simulink model "ForceBasedRollCenterModel"  (R2020b)
settings: Solver=VariableStepAuto  StartTime=0.0  StopTime=10.0  MaxStep=10E-2  RelTol=1e-3
settings Model: Creator=Authorized User  LastModifiedBy=Authorized User

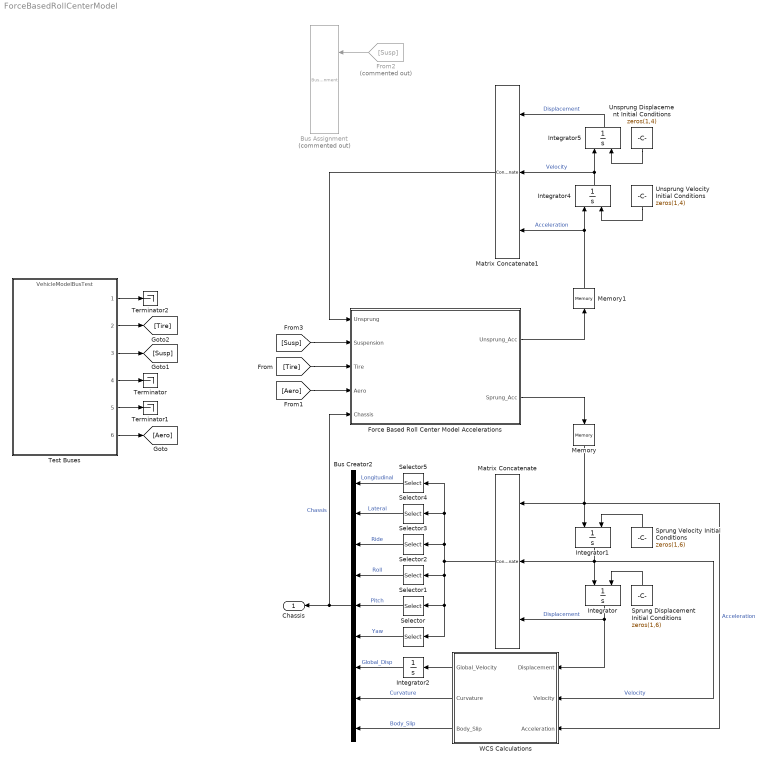
== system ForceBasedRollCenterModel ==
  Bus Assignment : BusAssignment  Commented=on  AssignedSignals=signal1
  Bus Creator2 : BusCreator  Inputs=9
  Force Based Roll Center Model Accelerations : MATLAB Function  TreatAsAtomicUnit=on
  From2 : From  Commented=on  GotoTag=Susp
  Integrator{,1,4..5} (4 alike) : Integrator  InitialConditionSource=external
  Integrator2 : Integrator
  Matrix Concatenate : Concatenate  NumInputs=3  Mode=Multidimensional array  ConcatenateDimension=2
  Matrix Concatenate1 : Concatenate  NumInputs=3  Mode=Multidimensional array  ConcatenateDimension=2
  Memory : Memory
  Memory1 : Memory
  Selector : Selector  NumberOfDimensions=2  InputPortWidth=3  IndexOptions=Index vector (dialog),Index vector (dialog)  Indices=6,[3 2 1]  OutputSizes=1,1
  Selector1 : Selector  NumberOfDimensions=2  InputPortWidth=3  IndexOptions=Index vector (dialog),Index vector (dialog)  Indices=5,[3 2 1]  OutputSizes=1,1
  Selector2 : Selector  NumberOfDimensions=2  InputPortWidth=3  IndexOptions=Index vector (dialog),Index vector (dialog)  Indices=4,[3 2 1]  OutputSizes=1,1
  Selector3 : Selector  NumberOfDimensions=2  InputPortWidth=3  IndexOptions=Index vector (dialog),Index vector (dialog)  Indices=3,[3 2 1]  OutputSizes=1,1
  Selector4 : Selector  NumberOfDimensions=2  InputPortWidth=3  IndexOptions=Index vector (dialog),Index vector (dialog)  Indices=2,[3 2 1]  OutputSizes=1,1
  Selector5 : Selector  NumberOfDimensions=2  InputPortWidth=3  IndexOptions=Index vector (dialog),Index vector (dialog)  Indices=1,[3 2 1]  OutputSizes=1,1
  Sprung Displacement Initial Conditions : Constant  Value=zeros(1,6)
  Sprung Velocity Initial Conditions : Constant  Value=zeros(1,6)
  Terminator : Terminator
  Terminator1 : Terminator
  Terminator2 : Terminator
  Test Buses : ModelReference  ModelNameDialog=VehicleModelBusTest.slx  SimulationMode=Normal  ModelReferenceVersion=1.30
  Unsprung Displacement Initial Conditions : Constant  Value=zeros(1,4)
  Unsprung Velocity Initial Conditions : Constant  Value=zeros(1,4)
  WCS Calculations : MATLAB Function  TreatAsAtomicUnit=on
  Chassis : Outport  OutDataTypeStr=Bus: Chassis
  wires:
  Test Buses/4 -> Terminator/1
  Test Buses/5 -> Terminator1/1
  Bus Creator2/1 -> Chassis/1, Force Based Roll Center Model Accelerations/5(Chassis)  "Chassis"
  Matrix Concatenate/1 -> Selector5/1, Selector4/1, Selector3/1, Selector/1, Selector1/1, Selector2/1
  Integrator1/1 -> Integrator/1, WCS Calculations/2(Velocity), Matrix Concatenate/2  "Velocity"
  Integrator/1 -> WCS Calculations/1(Displacement), Matrix Concatenate/3  "Displacement"
  WCS Calculations/2(Curvature) -> Bus Creator2/8  "Curvature"
  WCS Calculations/3(Body_Slip) -> Bus Creator2/9  "Body_Slip"
  WCS Calculations/1(Global_Velocity) -> Integrator2/1
  Selector/1 -> Bus Creator2/6  "Yaw"
  Selector1/1 -> Bus Creator2/5  "Pitch"
  Selector2/1 -> Bus Creator2/4  "Roll"
  Selector3/1 -> Bus Creator2/3  "Ride"
  Selector4/1 -> Bus Creator2/2  "Lateral"
  Selector5/1 -> Bus Creator2/1  "Longitudinal"
  Test Buses/1 -> Terminator2/1
  Sprung Velocity Initial Conditions/1 -> Integrator1/2
  Sprung Displacement Initial Conditions/1 -> Integrator/2
  Integrator2/1 -> Bus Creator2/7  "Global_Disp"
  Memory/1 -> Integrator1/1, WCS Calculations/3(Acceleration), Matrix Concatenate/1  "Acceleration"
  Force Based Roll Center Model Accelerations/2(Sprung_Acc) -> Memory/1
  Integrator4/1 -> Matrix Concatenate1/2, Integrator5/1  "Velocity"
  Integrator5/1 -> Matrix Concatenate1/1  "Displacement"
  Force Based Roll Center Model Accelerations/1(Unsprung_Acc) -> Memory1/1
  Unsprung Velocity Initial Conditions/1 -> Integrator4/2
  Unsprung Displacement Initial Conditions/1 -> Integrator5/2
  Test Buses/6 -> [Aero]
  Test Buses/2 -> [Tire]
  Test Buses/3 -> [Susp]
  [Tire] -> Force Based Roll Center Model Accelerations/3(Tire)
  [Aero] -> Force Based Roll Center Model Accelerations/4(Aero)
  From2/1 -> Bus Assignment/1
  [Susp] -> Force Based Roll Center Model Accelerations/2(Suspension)
  Matrix Concatenate1/1 -> Force Based Roll Center Model Accelerations/1(Unsprung)
  Memory1/1 -> Integrator4/1, Matrix Concatenate1/3  "Acceleration"

== matlab function ForceBasedRollCenterModel/WCS Calculations ==
  data: Displacement input; Velocity input; Global_Velocity output; Curvature output; Body_Slip output; Acceleration input
function [Global_Velocity, Curvature, Body_Slip] = ...
    WCS_Calculations( Displacement, Velocity, Acceleration )
%% Nomenclature
% Yaw Angle                : Displacement(6)
% Longitudinal Velocity    : Velocity(1) 
% Longitudinal Acceleration: Acceleration(1)
% Lateral Velocity         : Velocity(2) 
% Lateral Acceleration     : Acceleration(2)

%% Global Displacement
Global_Velocity = zeros(1,2);

Global_Velocity(1) = Velocity(1) .* cosd( Displacement(6) ) - ...
                     Velocity(2) .* sind( Displacement(6) );
                 
Global_Velocity(2) = Velocity(1) .* sind( Displacement(6) ) + ...
                     Velocity(2) .* cosd( Displacement(6) );  
                 
%% Curvature
if abs(Velocity(1).^2 + Velocity(2).^2) <= 0.01
    Curvature = 1000;
else
    Curvature = abs( Acceleration(1).*Velocity(2) - Velocity(1).*Acceleration(2) ) ./ ...
        ( Velocity(2).^2 + Velocity(2).^2 ).^(3/2);
end

%% Body Slip
Body_Slip = atan2d( Velocity(2), Velocity(1) );

== matlab function ForceBasedRollCenterModel/Force Based Roll Center Model Accelerations ==
  data: Unsprung input; Suspension input; Tire input; Aero input; Chassis input; Unsprung_Acc output; Sprung_Acc output
function [Unsprung_Acc, Sprung_Acc] = ...
    Acceleration_Evaluation( Unsprung, Suspension, Tire, Aero, Chassis )
%% Initialization
Unsprung_Acc = ones(4,1);
Sprung_Acc = zeros(6,1);

%% Sprung Dynamics
%%% Longitudinal Dynamics
Sprung_Acc(1) = 1;

%%% Lateral Dynamics
Sprung_Acc(2) = 1;

%%% Ride Dynamics
Sprung_Acc(3) = 1;

%%% Roll Dynamics
Sprung_Acc(4) = 0;

%%% Pitch Dynamics
Sprung_Acc(5) = 1;

%%% Yaw Dynamics
Sprung_Acc(6) = 1;
